simulink model "single_tank_linear_known_disturbance_real_PID"  (R2022a)
settings: Solver=VariableStepAuto  StartTime=0.0  StopTime=10.0  RelTol=1e-3
values from neighbouring files (symbols this model uses):
  dt = 1    [linear_version_known_disturbance_real_PID.m]
  h_0 = 30    [state_space_models.m]
  I_0 = [ 0 0 0 ]    [state_space_models.m]
  K_noise = 0*196*10^(-4)    (= 0)    [linear_version_known_disturbance_real_PID.m]
  MPC_active = 1    [linear_version_known_disturbance_real_PID.m]
  sys_kd = c2d(ss(A_kc,B_kc,C_kc,D_kc), dt)    [state_space_models.m]
  sys_pd = c2d(ss(A_pc,[B_pc B_pc_d],C_pc,D_pc), dt)    [state_space_models.m]
  u_0 = 60    [state_space_models.m]
  x_0 = 0    [state_space_models.m]
undefined symbols (not defined in the file or in its folder): dist
libraries: mpclib x1
settings Model: Creator=100238  LastModifiedBy=100238

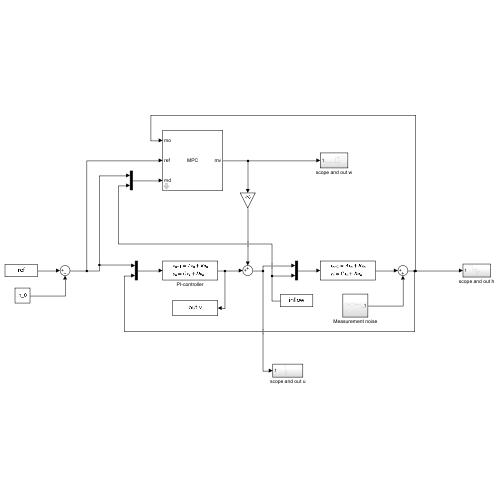
[thumbnail: Simulink's stored preview of the top-level diagram]
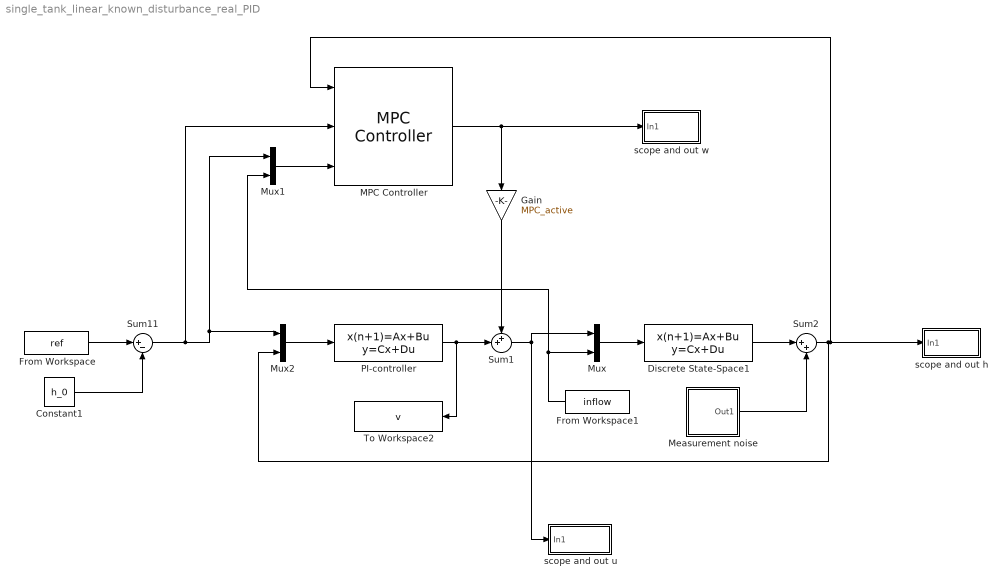
== system single_tank_linear_known_disturbance_real_PID ==
  Constant1 : Constant  Value=h_0
  Discrete State-Space1 : DiscreteStateSpace  A=sys_pd.A  B=sys_pd.B  C=sys_pd.C  D=sys_pd.D  InitialCondition=x_0  SampleTime=dt
  From Workspace : FromWorkspace  VariableName=ref  SampleTime=dt
  From Workspace1 : FromWorkspace  VariableName=inflow  SampleTime=dt
  Gain : Gain  Gain=MPC_active
  MPC Controller : mpclib/MPC Controller  SCDEnableBlockLinearizationSpecification=on  mpcobj=mpc_controller  is_multiple=0  enable_value=0  return_u0=off  updateMPCinCallerWorkspace=on  md_inport=on  mv_inport=off  uref_inport=off  return_cost=off  return_mvseq=off  return_qpstatus=off  return_xseq=off  return_state=off  return_ovseq=off  state_inport=off  umin_inport=off  umax_inport=off  ymin_inport=off  ymax_inport=off  cc_inport=off  ywt_inport=off  uwt_inport=off  duwt_inport=off  rhoeps_inport=off  pm_inport=off  MaximumP=10  HorizonChoice=FixedHorizon  n_ts=1  n_p=150  n_mv=1  n_md=2  n_ud=0  n_mo=1  n_uo=0  BlockDataType=double  SampleTimeInherited=off  switch_inport=off
  Measurement noise : Subsystem
  Mux : Mux  Inputs=2
  Mux1 : Mux  Inputs=2
  Mux2 : Mux  Inputs=2
  PI-controller : DiscreteStateSpace  A=sys_kd.A  B=sys_kd.B  C=sys_kd.C  D=sys_kd.D  InitialCondition=I_0  SampleTime=dt
  Sum1 : Sum  Inputs=++|
  Sum11 : Sum  Inputs=|+-
  Sum2 : Sum  Inputs=|++
  To Workspace2 : ToWorkspace  VariableName=v  SampleTime=dt
  scope and out h : Subsystem
  scope and out u : Subsystem
  scope and out w : Subsystem
  wires:
  From Workspace1/1 -> Mux/2, Mux1/2
  Sum11/1 -> MPC Controller/2, Mux1/1, Mux2/1
  From Workspace/1 -> Sum11/1
  Constant1/1 -> Sum11/2
  Sum1/1 -> scope and out u/1(In1), Mux/1
  PI-controller/1 -> To Workspace2/1, Sum1/2
  Mux2/1 -> PI-controller/1
  MPC Controller/1 -> Gain/1, scope and out w/1(In1)
  Mux/1 -> Discrete State-Space1/1
  Mux1/1 -> MPC Controller/3
  Measurement noise/1(Out1) -> Sum2/2
  Discrete State-Space1/1 -> Sum2/1
  Sum2/1 -> MPC Controller/1, scope and out h/1(In1), Mux2/2
  Gain/1 -> Sum1/1

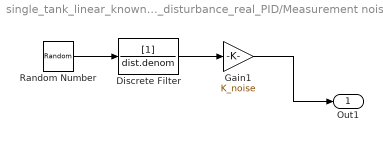
== system single_tank_linear_known_disturbance_real_PID/Measurement noise ==
  Discrete Filter : DiscreteFilter  Denominator=dist.denom  SampleTime=dt
  Gain1 : Gain  Gain=K_noise
  Random Number : RandomNumber  Seed=1  SampleTime=dt
  Out1 : Outport
  wires:
  Random Number/1 -> Discrete Filter/1
  Gain1/1 -> Out1/1
  Discrete Filter/1 -> Gain1/1

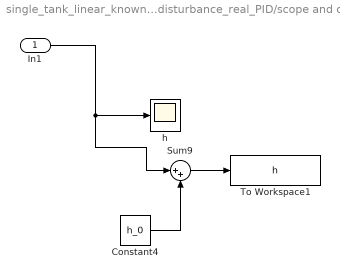
== system single_tank_linear_known_disturbance_real_PID/scope and out h ==
  In1 : Inport
  Constant4 : Constant  Value=h_0
  Sum9 : Sum  Inputs=|++
  To Workspace1 : ToWorkspace  VariableName=h  SampleTime=dt
  h : Scope
  wires:
  Sum9/1 -> To Workspace1/1
  In1/1 -> Sum9/1, h/1
  Constant4/1 -> Sum9/2

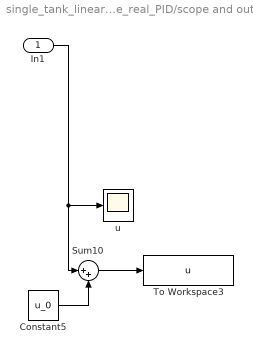
== system single_tank_linear_known_disturbance_real_PID/scope and out u ==
  In1 : Inport
  Constant5 : Constant  Value=u_0
  Sum10 : Sum  Inputs=|++
  To Workspace3 : ToWorkspace  VariableName=u  SampleTime=dt
  u : Scope
  wires:
  Constant5/1 -> Sum10/2
  Sum10/1 -> To Workspace3/1
  In1/1 -> u/1, Sum10/1

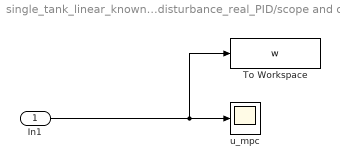
== system single_tank_linear_known_disturbance_real_PID/scope and out w ==
  In1 : Inport
  To Workspace : ToWorkspace  VariableName=w  SampleTime=dt
  u_mpc : Scope
  wires:
  In1/1 -> To Workspace/1, u_mpc/1
